simulink library "InterModuleProtocol"  (R2023b)
settings: Solver=VariableStepAuto  StartTime=0.0  StopTime=10.0  RelTol=1e-3
undefined symbols (not defined in the file or in its folder): accelerationNED, accelerationNEDXYZ, accelerationXYZ, angleOfAttack, courseOverGround, orientationQuaternion, orientationRollPitchYaw, positionLLA, positionNED, sideSlipAngle, speedOverGround, velocityNED, velocityNEDUVW, velocityPQR, velocityUVW
libraries: $bdroot x10
(part 1 of 3)
settings Model: Creator=Scythe  LastModifiedBy=Scythe
settings SolverCC: AlgebraicLoopSolver=TrustRegion
settings DataIOCC: ReturnWorkspaceOutputs=off
settings OptimizationCC: ReuseModelBlockBuffer=off
settings DebuggingCC: UnconnectedInputMsg=warning  UnconnectedOutputMsg=warning  UnconnectedLineMsg=warning  ArithmeticOperatorsInVariantConditions=warning
settings ModelReferenceCC: EnableRefExpFcnMdlSchedulingChecks=on
settings SFSimCC: CustomCodeUndefinedFunction=UseInterfaceOnly
settings RTWCC: DLArmComputeVersion=19.05

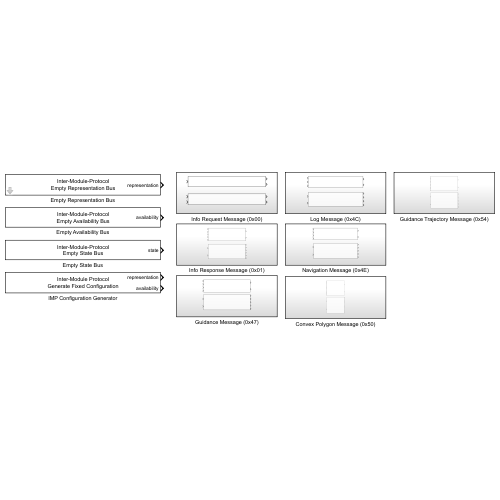
[thumbnail: Simulink's stored preview of the top-level diagram]
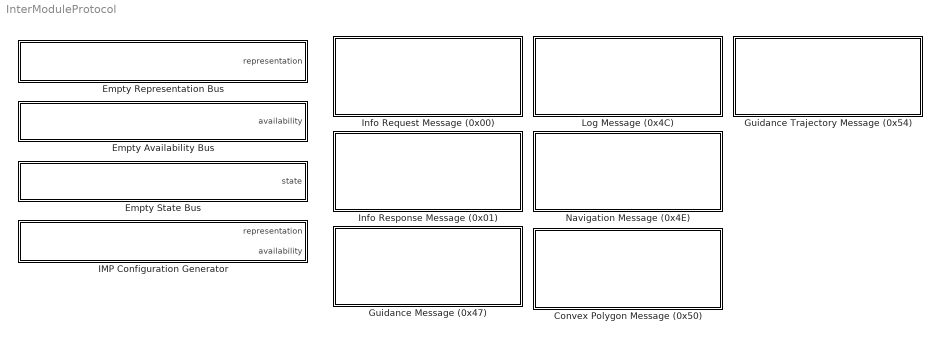
== system InterModuleProtocol ==
  Convex Polygon Message (0x50) : Subsystem
  Empty Availability Bus : Subsystem
      mask help: Create an empty availability bus for the Inter-Module Protocol (IMP). All values inside the bus are zero.
      mask DialogControl DescGroupVar Prompt: Empty Availability Bus
      mask Display: disp('Inter-Module-Protocol\nEmpty Availability Bus');
  Empty Representation Bus : Subsystem
      mask help: Create an empty representation bus for the Inter-Module Protocol (IMP). All values inside the bus are zero.
      mask DialogControl DescGroupVar Prompt: Empty Representation Bus
      mask Display: disp('Inter-Module-Protocol\nEmpty Representation Bus');
  Empty State Bus : Subsystem
      mask help: Create an empty state bus for the Inter-Module Protocol (IMP). All values inside the bus are zero. However, the scalar part of the quaternion is set to one.
      mask DialogControl DescGroupVar Prompt: Empty State Bus
      mask Display: disp('Inter-Module-Protocol\nEmpty State Bus');
  Guidance Message (0x47) : Subsystem
  Guidance Trajectory Message (0x54) : Subsystem
  IMP Configuration Generator : Subsystem  mask{positionLLAAvailability=0 DoF - none, positionLLARepresentation=8 bytes (double), positionNEDAvailability=0 DoF - none, positionNEDRepresentation=8 bytes (double), orientationQuaternionAvailability=0 DoF - none, orientationQuaternionRepresentation=8 bytes (double), orientationRPYAvailability=0 DoF - none, orientationRPYRepresentation=8 bytes (double), velocityNEDUVWAvailabilityE=0 DoF - none, velocityNEDUVWAvailabilityB=0 DoF - none, velocityNEDUVWRepresentation=8 bytes (double), velocityPQRAvailability=0 DoF - none, velocityPQRRepresentation=8 bytes (double), accelerationNEDXYZAvailabilityE=0 DoF - none, accelerationNEDXYZAvailabilityB=0 DoF - none, accelerationNEDXYZRepresentation=8 bytes (double), courseOverGroundAvailability=0 - disable, courseOverGroundRepresentation=8 bytes (double), speedOverGroundAvailability=0 - disable, speedOverGroundRepresentation=8 bytes (double), angleOfAttackAvailability=0 - disable, angleOfAttackRepresentation=8 bytes (double), sideSlipAngleAvailability=0 - disable, sideSlipAngleRepresentation=8 bytes (double)}
      mask prompts: positionLLAAvailability "Position (latitude, longitude, altitude):"; positionLLARepresentation ""; positionNEDAvailability "Position (NED):"; positionNEDRepresentation ""; orientationQuaternionAvailability "Orientation (quaternion):"; orientationQuaternionRepresentation ""; orientationRPYAvailability "Orientation (roll, pitch, yaw):"; orientationRPYRepresentation ""; velocityNEDUVWAvailabilityE "Velocity (NED, uvw):"; velocityPQRAvailability "Velocity (pqr):"; velocityPQRRepresentation ""; accelerationNEDXYZAvailabilityE "Acceleration (NED, XYZ):"; courseOverGroundAvailability "Course over ground:"; courseOverGroundRepresentation ""; speedOverGroundAvailability "Speed over ground:"; speedOverGroundRepresentation ""; angleOfAttackAvailability "Angle of attack:"; angleOfAttackRepresentation ""; sideSlipAngleAvailability "Side slip angle:"; sideSlipAngleRepresentation ""
      mask help: Generate a fixed configuration (representation and availability) to be used for encoding messages like navigation and guidance messages. The configuration is used to encode a variable-data message. For each value in a message, select the degree of freedom (DoF) and the data type representation to be encoded.
      mask TypeOptions positionLLAAvailability: 0 DoF - none | 1 DoF - alt | 2 DoF - lat, lon | 3 DoF - lat, lon, alt
      mask TypeOptions positionLLARepresentation: 4 bytes (int32, float) | 8 bytes (double)
      mask TypeOptions positionNEDAvailability: 0 DoF - none | 1 DoF - down | 2 DoF - north, east | 3 DoF - north, east, down
      mask TypeOptions positionNEDRepresentation: 4 bytes (float) | 8 bytes (double)
      mask TypeOptions orientationQuaternionAvailability: 0 DoF - none | 3 DoF - qw, qx, qy, qz
      mask TypeOptions orientationQuaternionRepresentation: 4 bytes (int32) | 8 bytes (double)
      mask TypeOptions orientationRPYAvailability: 0 DoF - none | 1 DoF - yaw | 2 DoF - roll, pitch | 3 DoF - roll, pitch, yaw
      mask TypeOptions orientationRPYRepresentation: 4 bytes (int32) | 8 bytes (double)
      mask TypeOptions velocityNEDUVWAvailabilityE: 0 DoF - none | 1 DoF - down | 2 DoF - north, east | 3 DoF - north, east, down
      mask TypeOptions velocityNEDUVWAvailabilityB: 0 DoF - none | 1 DoF - w | 2 DoF - u, v | 3 DoF - u, v, w
      mask TypeOptions velocityNEDUVWRepresentation: 4 bytes (float) | 8 bytes (double)
      mask TypeOptions velocityPQRAvailability: 0 DoF - none | 1 DoF - r | 2 DoF - p, q | 3 DoF - p, q, r
      mask TypeOptions velocityPQRRepresentation: 4 bytes (float) | 8 bytes (double)
      mask TypeOptions accelerationNEDXYZAvailabilityE: 0 DoF - none | 1 DoF - down | 2 DoF - north, east | 3 DoF - north, east, down
      mask TypeOptions accelerationNEDXYZAvailabilityB: 0 DoF - none | 1 DoF - Z | 2 DoF - X, Y | 3 DoF - X, Y, Z
      mask TypeOptions accelerationNEDXYZRepresentation: 4 bytes (float) | 8 bytes (double)
      mask TypeOptions courseOverGroundAvailability: 0 - disable | 1 - enable
      mask TypeOptions courseOverGroundRepresentation: 4 bytes (int32) | 8 bytes (double)
      mask TypeOptions speedOverGroundAvailability: 0 - disable | 1 - enable
      mask TypeOptions speedOverGroundRepresentation: 4 bytes (float) | 8 bytes (double)
      mask TypeOptions angleOfAttackAvailability: 0 - disable | 1 - enable
      mask TypeOptions angleOfAttackRepresentation: 4 bytes (int32) | 8 bytes (double)
      mask TypeOptions sideSlipAngleAvailability: 0 - disable | 1 - enable
      mask TypeOptions sideSlipAngleRepresentation: 4 bytes (int32) | 8 bytes (double)
      mask DialogControl DescGroupVar Prompt: Generate Fixed Configuration
      mask DialogControl ParameterGroupVar Prompt: Configuration
      mask Display: disp('Inter-Module Protocol\nGenerate Fixed Configuration');
  Info Request Message (0x00) : Subsystem
  Info Response Message (0x01) : Subsystem
  Log Message (0x4C) : Subsystem
  Navigation Message (0x4E) : Subsystem

== system InterModuleProtocol/Convex Polygon Message (0x50) ==
  Decode Convex Polygon Message : Subsystem  mask{maxNumPolygons=10}
      mask prompts: maxNumPolygons "Maximum number of polygons:"
      mask help:
      | Decode a convex polygon message (Inter-Module Protocol).<br><br>
      |
      | <b>numDecodedBytes</b><br>Number of decoded bytes (negative value if error occurred).<br><br>
      | <b>timestampUTC</b><br>UTC second of the day.<br><br>
      | <b>maxSegmentIndex</b><br>The maximum zero-based segment index that indicates the last message segment. That is, the maximum number of polgon messages belonging to a polygon dataset is (maxSegmentIndex + 1).<br><br>
      | <b>segmentIndex</b><br>The current zero-based segment index for this message.<br><br>
      | <b>originLLA</b><br>Latitude [rad], longitude [rad] and altitude [m] of the origin.<br><br>
      | <b>polygons</b><br>A 2-by-255-by-np matrix containing the vertices for all polygons (column-major order) with np being the maximum number of polygons. A vertex consists of two elements (x and y).<br><br>
      | <b>numVertices</b><br>An np-by-1 vector containing the unique IDs for all polygons in the polygon matrix.<br><br>
      | <b>polygonIDs</b><br>An np-by-1 vector containing the unique IDs for all polygons in the polygon matrix with np being the maximum number of polygons.<br><br>
      | <b>classifications</b><br>An np-by-1 vector containing the classifications for all polygons in the polygon matrix with np being the maximum number of polygons.<br><br>
      | <b>velocitiesNorth</b><br>An np-by-1 vector containing the north velocities in meters per second for all polygons in the polygon matrix with np being the maximum number of polygons. All velocities of a polygon refer to the mean value of all vertices of this polygon.<br><br>
      | <b>velocitiesEast</b><br>An np-by-1 vector containing the east velocities in meters per second for all polygons in the polygon matrix with np being the maximum number of polygons. All velocities of a polygon refer to the mean value of all vertices of this polygon.<br><br>
      | <b>velocitiesYawRate</b><br>An np-by-1 vector containing the rotational rates of turn in radians per second for all polygons in the polygon matrix with np being the maximum number of polygons. All velocities of a polygon refer to the mean value of all vertices of this polygon.<br><br>
      | <b>numPolygons</b><br>The number of decoded polygons.
      mask Help: eval('IMP_OpenDocumentation(''#ConvexPolygonMessage'');');
      mask DialogControl DescGroupVar Prompt: Decode Convex Polygon Message
      mask Display: disp('Inter-Module-Protocol\nDecode Convex Polygon Message');
  Encode Convex Polygon Message : Subsystem  mask{outBufferSize=1024, maxNumPolygons=10}
      mask prompts: outBufferSize "Output buffer size:"; maxNumPolygons "Maximum number of polygons:"
      mask help:
      | Encode a convex polygon message (Inter-Module Protocol).<br><br>
      |
      | <b>timestampUTC</b><br>UTC second of the day.<br><br>
      | <b>maxSegmentIndex</b><br>The maximum zero-based segment index that indicates the last message segment. That is, the maximum number of polgon messages belonging to a polygon dataset is (maxSegmentIndex + 1).<br><br>
      | <b>segmentIndex</b><br>The current zero-based segment index for this message.<br><br>
      | <b>originLLA</b><br>Latitude [rad], longitude [rad] and altitude [m] of the origin.<br><br>
      | <b>polygons</b><br>A 2-by-255-by-np matrix containing the vertices for all polygons (column-major order) with np being the maximum number of polygons. A vertex consists of two elements (x and y).<br><br>
      | <b>numVertices</b><br>An np-by-1 vector containing the actual number of vertices per polygon in the polygon matrix.<br><br>
      | <b>polygonIDs</b><br>An np-by-1 vector containing the unique IDs for all polygons in the polygon matrix with np being the maximum number of polygons.<br><br>
      | <b>classifications</b><br>An np-by-1 vector containing the classifications for all polygons in the polygon matrix with np being the maximum number of polygons.<br><br>
      | <b>velocitiesNorth</b><br>An np-by-1 vector containing the north velocities in meters per second for all polygons in the polygon matrix with np being the maximum number of polygons. All velocities of a polygon refer to the mean value of all vertices of this polygon.<br><br>
      | <b>velocitiesEast</b><br>An np-by-1 vector containing the east velocities in meters per second for all polygons in the polygon matrix with np being the maximum number of polygons. All velocities of a polygon refer to the mean value of all vertices of this polygon.<br><br>
      | <b>velocitiesYawRate</b><br>An np-by-1 vector containing the rotational rates of turn in radians per second for all polygons in the polygon matrix with np being the maximum number of polygons. All velocities of a polygon refer to the mean value of all vertices of this polygon.<br><br>
      | <b>numPolygons</b><br>The number of polygons to be used for encoding.
      mask Help: eval('IMP_OpenDocumentation(''#ConvexPolygonMessage'');');
      mask DialogControl DescGroupVar Prompt: Encode Convex Polygon Message
      mask Display: disp('Inter-Module-Protocol\nEncode Convex Polygon Message');

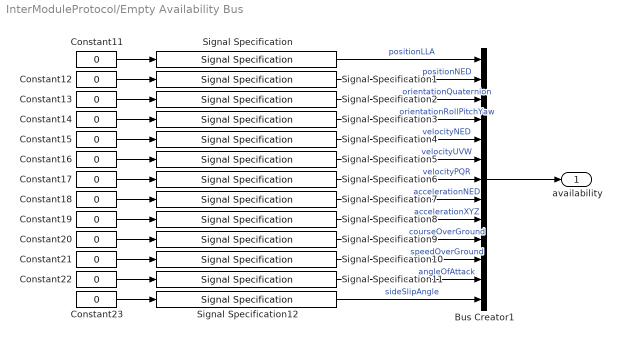
== system InterModuleProtocol/Empty Availability Bus ==
  Bus Creator1 : BusCreator  Inputs=13
  Constant{11..23} (13 alike) : Constant  Value=0  OutDataTypeStr=uint8
  Signal Specification{,1..12} (13 alike) : SignalSpecification  OutDataTypeStr=uint8  Dimensions=1
  availability : Outport  VectorParamsAs1DForOutWhenUnconnected=off
  wires:
  Signal Specification10/1 -> Bus Creator1/11  "speedOverGround"
  Signal Specification3/1 -> Bus Creator1/4  "orientationRollPitchYaw"
  Signal Specification4/1 -> Bus Creator1/5  "velocityNED"
  Signal Specification12/1 -> Bus Creator1/13  "sideSlipAngle"
  Bus Creator1/1 -> availability/1
  Signal Specification1/1 -> Bus Creator1/2  "positionNED"
  Signal Specification9/1 -> Bus Creator1/10  "courseOverGround"
  Signal Specification5/1 -> Bus Creator1/6  "velocityUVW"
  Signal Specification6/1 -> Bus Creator1/7  "velocityPQR"
  Signal Specification2/1 -> Bus Creator1/3  "orientationQuaternion"
  Signal Specification/1 -> Bus Creator1/1  "positionLLA"
  Signal Specification7/1 -> Bus Creator1/8  "accelerationNED"
  Signal Specification8/1 -> Bus Creator1/9  "accelerationXYZ"
  Signal Specification11/1 -> Bus Creator1/12  "angleOfAttack"
  Constant11/1 -> Signal Specification/1
  Constant12/1 -> Signal Specification1/1
  Constant13/1 -> Signal Specification2/1
  Constant14/1 -> Signal Specification3/1
  Constant15/1 -> Signal Specification4/1
  Constant16/1 -> Signal Specification5/1
  Constant23/1 -> Signal Specification12/1
  Constant22/1 -> Signal Specification11/1
  Constant21/1 -> Signal Specification10/1
  Constant20/1 -> Signal Specification9/1
  Constant19/1 -> Signal Specification8/1
  Constant18/1 -> Signal Specification7/1
  Constant17/1 -> Signal Specification6/1

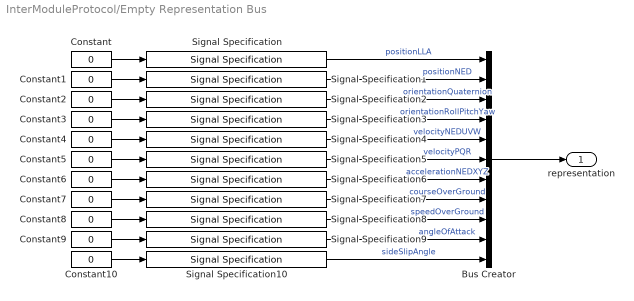
== system InterModuleProtocol/Empty Representation Bus ==
  Bus Creator : BusCreator  Inputs=11
  Constant{,1..10} (11 alike) : Constant  Value=0  OutDataTypeStr=uint8
  Signal Specification{,1..10} (11 alike) : SignalSpecification  OutDataTypeStr=uint8  Dimensions=1
  representation : Outport  VectorParamsAs1DForOutWhenUnconnected=off
  wires:
  Signal Specification10/1 -> Bus Creator/11  "sideSlipAngle"
  Signal Specification1/1 -> Bus Creator/2  "positionNED"
  Signal Specification8/1 -> Bus Creator/9  "speedOverGround"
  Bus Creator/1 -> representation/1
  Signal Specification9/1 -> Bus Creator/10  "angleOfAttack"
  Signal Specification7/1 -> Bus Creator/8  "courseOverGround"
  Signal Specification6/1 -> Bus Creator/7  "accelerationNEDXYZ"
  Signal Specification4/1 -> Bus Creator/5  "velocityNEDUVW"
  Signal Specification5/1 -> Bus Creator/6  "velocityPQR"
  Signal Specification3/1 -> Bus Creator/4  "orientationRollPitchYaw"
  Signal Specification2/1 -> Bus Creator/3  "orientationQuaternion"
  Signal Specification/1 -> Bus Creator/1  "positionLLA"
  Constant/1 -> Signal Specification/1
  Constant1/1 -> Signal Specification1/1
  Constant2/1 -> Signal Specification2/1
  Constant3/1 -> Signal Specification3/1
  Constant4/1 -> Signal Specification4/1
  Constant5/1 -> Signal Specification5/1
  Constant6/1 -> Signal Specification6/1
  Constant7/1 -> Signal Specification7/1
  Constant8/1 -> Signal Specification8/1
  Constant9/1 -> Signal Specification9/1
  Constant10/1 -> Signal Specification10/1

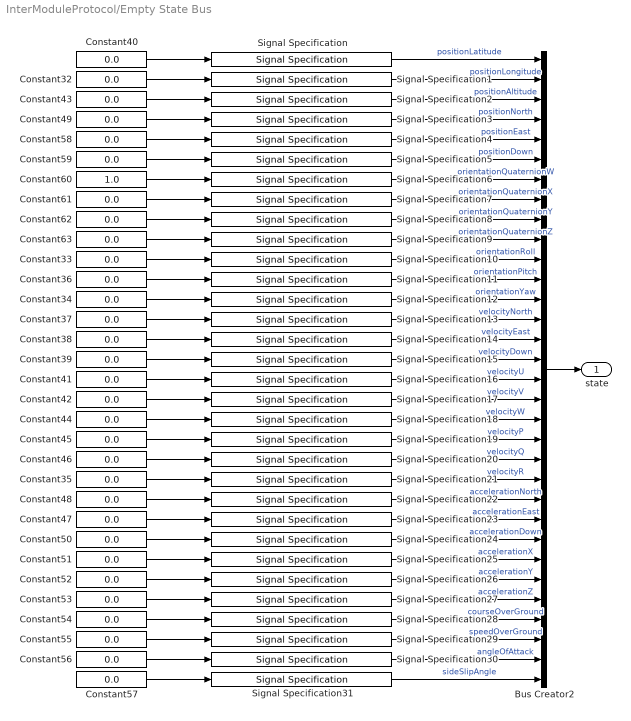
== system InterModuleProtocol/Empty State Bus ==
  Bus Creator2 : BusCreator  Inputs=32
  Constant{32..59,61..63} (31 alike) : Constant  Value=0.0
  Constant60 : Constant  Value=1.0
  Signal Specification{,1,10..12,28,30..31} (8 alike) : SignalSpecification  OutDataTypeStr=double  Unit=rad  Dimensions=1
  Signal Specification{13..18,29} (7 alike) : SignalSpecification  OutDataTypeStr=double  Unit=m/s  Dimensions=1
  Signal Specification19 : SignalSpecification  OutDataTypeStr=double  Unit=rad/s  Dimensions=1
  Signal Specification{2..5} (4 alike) : SignalSpecification  OutDataTypeStr=double  Unit=m  Dimensions=1
  Signal Specification20 : SignalSpecification  OutDataTypeStr=double  Unit=rad/s  Dimensions=1
  Signal Specification21 : SignalSpecification  OutDataTypeStr=double  Unit=rad/s  Dimensions=1
  Signal Specification{22..27} (6 alike) : SignalSpecification  OutDataTypeStr=double  Unit=m/s^2  Dimensions=1
  Signal Specification{6..9} (4 alike) : SignalSpecification  OutDataTypeStr=double  Dimensions=1
  state : Outport  VectorParamsAs1DForOutWhenUnconnected=off
  wires:
  Signal Specification29/1 -> Bus Creator2/30  "speedOverGround"
  Signal Specification2/1 -> Bus Creator2/3  "positionAltitude"
  Signal Specification8/1 -> Bus Creator2/9  "orientationQuaternionY"
  Signal Specification17/1 -> Bus Creator2/18  "velocityV"
  Bus Creator2/1 -> state/1
  Signal Specification25/1 -> Bus Creator2/26  "accelerationX"
  Signal Specification1/1 -> Bus Creator2/2  "positionLongitude"
  Signal Specification27/1 -> Bus Creator2/28  "accelerationZ"
  Signal Specification3/1 -> Bus Creator2/4  "positionNorth"
  Signal Specification12/1 -> Bus Creator2/13  "orientationYaw"
  Signal Specification18/1 -> Bus Creator2/19  "velocityW"
  Signal Specification24/1 -> Bus Creator2/25  "accelerationDown"
  Signal Specification22/1 -> Bus Creator2/23  "accelerationNorth"
  Signal Specification/1 -> Bus Creator2/1  "positionLatitude"
  Signal Specification15/1 -> Bus Creator2/16  "velocityDown"
  Signal Specification14/1 -> Bus Creator2/15  "velocityEast"
  Signal Specification10/1 -> Bus Creator2/11  "orientationRoll"
  Signal Specification26/1 -> Bus Creator2/27  "accelerationY"
  Signal Specification30/1 -> Bus Creator2/31  "angleOfAttack"
  Signal Specification6/1 -> Bus Creator2/7  "orientationQuaternionW"
  Signal Specification13/1 -> Bus Creator2/14  "velocityNorth"
  Signal Specification11/1 -> Bus Creator2/12  "orientationPitch"
  Signal Specification16/1 -> Bus Creator2/17  "velocityU"
  Signal Specification21/1 -> Bus Creator2/22  "velocityR"
  Signal Specification19/1 -> Bus Creator2/20  "velocityP"
  Signal Specification31/1 -> Bus Creator2/32  "sideSlipAngle"
  Signal Specification4/1 -> Bus Creator2/5  "positionEast"
  Signal Specification7/1 -> Bus Creator2/8  "orientationQuaternionX"
  Signal Specification5/1 -> Bus Creator2/6  "positionDown"
  Signal Specification9/1 -> Bus Creator2/10  "orientationQuaternionZ"
  Signal Specification28/1 -> Bus Creator2/29  "courseOverGround"
  Signal Specification20/1 -> Bus Creator2/21  "velocityQ"
  Signal Specification23/1 -> Bus Creator2/24  "accelerationEast"
  Constant50/1 -> Signal Specification24/1
  Constant56/1 -> Signal Specification30/1
  Constant52/1 -> Signal Specification26/1
  Constant47/1 -> Signal Specification23/1
  Constant33/1 -> Signal Specification10/1
  Constant43/1 -> Signal Specification2/1
  Constant40/1 -> Signal Specification/1
  Constant51/1 -> Signal Specification25/1
  Constant34/1 -> Signal Specification12/1
  Constant49/1 -> Signal Specification3/1
  Constant36/1 -> Signal Specification11/1
  Constant37/1 -> Signal Specification13/1
  Constant35/1 -> Signal Specification21/1
  Constant55/1 -> Signal Specification29/1
  Constant62/1 -> Signal Specification8/1
  Constant63/1 -> Signal Specification9/1
  Constant54/1 -> Signal Specification28/1
  Constant53/1 -> Signal Specification27/1
  Constant39/1 -> Signal Specification15/1
  Constant59/1 -> Signal Specification5/1
  Constant41/1 -> Signal Specification16/1
  Constant61/1 -> Signal Specification7/1
  Constant38/1 -> Signal Specification14/1
  Constant58/1 -> Signal Specification4/1
  Constant60/1 -> Signal Specification6/1
  Constant46/1 -> Signal Specification20/1
  Constant32/1 -> Signal Specification1/1
  Constant44/1 -> Signal Specification18/1
  Constant57/1 -> Signal Specification31/1
  Constant42/1 -> Signal Specification17/1
  Constant48/1 -> Signal Specification22/1
  Constant45/1 -> Signal Specification19/1

== system InterModuleProtocol/Guidance Message (0x47) ==
  Decode Guidance Message : Subsystem
      mask help:
      | Decode a guidance message (Inter-Module Protocol).<br><br>
      |
      | <b>numDecodedBytes</b><br>Number of decoded bytes (negative value if error occurred).<br><br>
      | <b>timestampUTC</b><br>UTC second of the day.<br><br>
      | <b>representation</b><br>Representation bus containing the datatype representation for the state.<br><br>
      | <b>availability</b><br>Availability bus containing the availability flags for the state.<br><br>
      | <b>state</b><br>The state bus containing the decoded values.
      mask Help: eval('IMP_OpenDocumentation(''#GuidanceMessage'');');
      mask DialogControl DescGroupVar Prompt: Decode Guidance Message
      mask Display: disp('Inter-Module-Protocol\nDecode Guidance Message');
  Encode Guidance Message : Subsystem  mask{outputBufferSize=268}
      mask prompts: outputBufferSize "Output buffer size:"
      mask help:
      | Encode a guidance message (Inter-Module Protocol).<br><br>
      |
      | <b>timestampUTC</b><br>UTC second of the day.<br><br>
      | <b>representation</b><br>The representation bus containing the data type representation for the state.
      | <br><br>
      |
      | <b>availability</b><br>The availability bus containing the availability flags for the state.
      | <br><br>
      |
      | <b>state</b><br>The state bus containing the values to be encoded.
      mask Help: eval('IMP_OpenDocumentation(''#GuidanceMessage'');');
      mask DialogControl DescGroupVar Prompt: Encode Guidance Message
      mask DialogControl Container2 Prompt: Parameters
      mask Display: disp('Inter-Module-Protocol\nEncode Guidance Message');

== system InterModuleProtocol/Guidance Trajectory Message (0x54) ==
  Decode Guidance Trajectory Message : Subsystem  mask{maxNumPoints=10}
      mask prompts: maxNumPoints "Maximum number of points:"
      mask help:
      | Decode a guidance trajectory message (Inter-Module Protocol).<br><br>
      |
      | <b>numDecodedBytes</b><br>Number of decoded bytes (negative value if error occurred).<br><br>
      | <b>timestampUTC</b><br>UTC second of the day.<br><br>
      | <b>startTimeYearUTC</b><br>Start time for the trajectory: year (UTC).<br><br>
      | <b>startTimeMonthUTC</b><br>Start time for the trajectory: month (UTC), range [1, 12].<br><br>
      | <b>startTimeDayUTC</b><br>Start time for the trajectory: day (UTC), range [1, 31].<br><br>
      | <b>startTimeSecondsUTC</b><br>Start time for the trajectory: seconds of the day (UTC).<br><br>
      | <b>deltaTime</b><br>Time difference from one state point to another in seconds. If this value is set to zero, then each point indicates a waypoint.<br><br>
      | <b>representation</b><br>Representation bus containing the datatype representation for a point.<br><br>
      | <b>availability</b><br>Availability bus containing the availability flags for a point.<br><br>
      | <b>points</b><br>32-by-N matrix containing N state vectors. N is the maximum number of points. Each column of the matrix is as follows:
      | <br>[0]: positionLatitude (rad)
      | <br>[1]: positionLongitude (rad)
      | <br>[2]: positionAltitude (m)
      | <br>[3]: positionNorth (m)
      | <br>[4]: positionEast (m)
      | <br>[5]: positionDown (m)
      | <br>[6]: orientationQuaternionW
      | <br>[7]: orientationQuaternionX
      | <br>[8]: orientationQuaternionY
      | <br>[9]: orientationQuaternionZ
      | <br>[10]: orientationRoll (rad)
      | <br>[11]: orientationPitch (rad)
      | <br>[12]: orientationYaw (rad)
      | <br>[13]: velocityNorth (m/s)
      | <br>[14]: velocityEast (m/s)
      | <br>[15]: velocityDown (m/s)
      | <br>[16]: velocityU (m/s)
      | <br>[17]: velocityV (m/s)
      | <br>[18]: velocityW (m/s)
      | <br>[19]: velocityP (rad/s)
      | <br>[20]: velocityQ (rad/s)
      | <br>[21]: velocityR (rad/s)
      | <br>[22]: accelerationNorth (m/(s*s))
      | <br>[23]: accelerationEast (m/(s*s))
      | <br>[24]: accelerationDown (m/(s*s))
      | <br>[25]: accelerationX (m/(s*s))
      | <br>[26]: accelerationY (m/(s*s))
      | <br>[27]: accelerationZ (m/(s*s))
      | <br>[28]: courseOverGround (rad)
      | <br>[29]: speedOverGround (m/s)
      | <br>[30]: angleOfAttack (rad)
      | <br>[31]: sideSlipAngle (rad)
      | <br><br>
      | <b>numPoints</b><br>Actual number of decoded points inside the output matrix.
      mask Help: eval('IMP_OpenDocumentation(''#GuidanceTrajectoryMessage'');');
      mask DialogControl DescGroupVar Prompt: Decode Guidance Trajectory Message
      mask Display: disp('Inter-Module-Protocol\nDecode Guidance Trajectory Message');
  Encode Guidance Trajectory Message : Subsystem  mask{maxNumPoints=10, outputBufferSize=1024}
      mask prompts: maxNumPoints "Maximum number of points:"; outputBufferSize "Output buffer size:"
      mask help:
      | Encode a guidance trajectory message (Inter-Module Protocol).<br><br>
      |
      | <b>timestampUTC</b><br>UTC second of the day.<br><br>
      | <b>startTimeYearUTC</b><br>Start time for the trajectory: year (UTC).<br><br>
      | <b>startTimeMonthUTC</b><br>Start time for the trajectory: month (UTC), range [1, 12].<br><br>
      | <b>startTimeDayUTC</b><br>Start time for the trajectory: day (UTC), range [1, 31].<br><br>
      | <b>startTimeSecondsUTC</b><br>Start time for the trajectory: seconds of the day (UTC).<br><br>
      | <b>deltaTime</b><br>Time difference from one state point to another in seconds. If this value is set to zero, then each point indicates a waypoint.<br><br>
      | <b>representation</b><br>The representation bus containing the data type representation for a point.<br><br>
      | <b>availability</b><br>The availability bus containing the availability flags for a point.<br><br>
      | <b>points</b><br>32-by-N matrix containing N state vectors. N is the number of points. Each column of the matrix is as follows:
      | <br>[0]: positionLatitude (rad)
      | <br>[1]: positionLongitude (rad)
      | <br>[2]: positionAltitude (m)
      | <br>[3]: positionNorth (m)
      | <br>[4]: positionEast (m)
      | <br>[5]: positionDown (m)
      | <br>[6]: orientationQuaternionW
      | <br>[7]: orientationQuaternionX
      | <br>[8]: orientationQuaternionY
      | <br>[9]: orientationQuaternionZ
      | <br>[10]: orientationRoll (rad)
      | <br>[11]: orientationPitch (rad)
      | <br>[12]: orientationYaw (rad)
      | <br>[13]: velocityNorth (m/s)
      | <br>[14]: velocityEast (m/s)
      | <br>[15]: velocityDown (m/s)
      | <br>[16]: velocityU (m/s)
      | <br>[17]: velocityV (m/s)
      | <br>[18]: velocityW (m/s)
      | <br>[19]: velocityP (rad/s)
      | <br>[20]: velocityQ (rad/s)
      | <br>[21]: velocityR (rad/s)
      | <br>[22]: accelerationNorth (m/(s*s))
      | <br>[23]: accelerationEast (m/(s*s))
      | <br>[24]: accelerationDown (m/(s*s))
      | <br>[25]: accelerationX (m/(s*s))
      | <br>[26]: accelerationY (m/(s*s))
      | <br>[27]: accelerationZ (m/(s*s))
      | <br>[28]: courseOverGround (rad)
      | <br>[29]: speedOverGround (m/s)
      | <br>[30]: angleOfAttack (rad)
      | <br>[31]: sideSlipAngle (rad)
      mask Help: eval('IMP_OpenDocumentation(''#GuidanceTrajectoryMessage'');');
      mask DialogControl DescGroupVar Prompt: Encode Guidance Trajectory Message
      mask Display: disp('Inter-Module-Protocol\nEncode Guidance Trajectory Message');

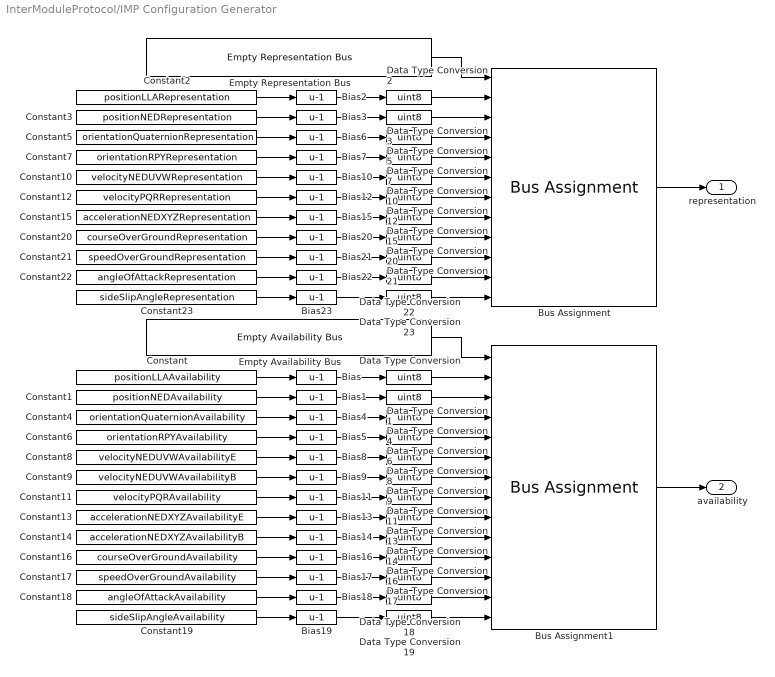
== system InterModuleProtocol/IMP Configuration Generator ==
  Bias{,1..23} (24 alike) : Bias  Bias=-1  SaturateOnIntegerOverflow=off
  Bus Assignment : BusAssignment  AssignedSignals=positionLLA,positionNED,orientationQuaternion,orientationRollPitchYaw,velocityNEDUVW,velocityPQR,accelerationNEDXYZ,courseOverGround,speedOverGround,angleOfAttack,sideSlipAngle
  Bus Assignment1 : BusAssignment  AssignedSignals=positionLLA,positionNED,orientationQuaternion,orientationRollPitchYaw,velocityNED,velocityUVW,velocityPQR,accelerationNED,accelerationXYZ,courseOverGround,speedOverGround,angleOfAttack,sideSlipAngle
  Constant : Constant  Value=positionLLAAvailability
  Constant1 : Constant  Value=positionNEDAvailability
  Constant10 : Constant  Value=velocityNEDUVWRepresentation
  Constant11 : Constant  Value=velocityPQRAvailability
  Constant12 : Constant  Value=velocityPQRRepresentation
  Constant13 : Constant  Value=accelerationNEDXYZAvailabilityE
  Constant14 : Constant  Value=accelerationNEDXYZAvailabilityB
  Constant15 : Constant  Value=accelerationNEDXYZRepresentation
  Constant16 : Constant  Value=courseOverGroundAvailability
  Constant17 : Constant  Value=speedOverGroundAvailability
  Constant18 : Constant  Value=angleOfAttackAvailability
  Constant19 : Constant  Value=sideSlipAngleAvailability
  Constant2 : Constant  Value=positionLLARepresentation
  Constant20 : Constant  Value=courseOverGroundRepresentation
  Constant21 : Constant  Value=speedOverGroundRepresentation
  Constant22 : Constant  Value=angleOfAttackRepresentation
  Constant23 : Constant  Value=sideSlipAngleRepresentation
  Constant3 : Constant  Value=positionNEDRepresentation
  Constant4 : Constant  Value=orientationQuaternionAvailability
  Constant5 : Constant  Value=orientationQuaternionRepresentation
  Constant6 : Constant  Value=orientationRPYAvailability
  Constant7 : Constant  Value=orientationRPYRepresentation
  Constant8 : Constant  Value=velocityNEDUVWAvailabilityE
  Constant9 : Constant  Value=velocityNEDUVWAvailabilityB
  Data Type Conversion{,1..23} (24 alike) : DataTypeConversion  OutDataTypeStr=uint8  SaturateOnIntegerOverflow=off  RndMeth=Floor
  Empty Availability Bus : $bdroot/Empty Availability Bus
  Empty Representation Bus : $bdroot/Empty Representation Bus
  representation : Outport
  availability : Outport  Port=2
  wires:
  Bias20/1 -> Data Type Conversion20/1
  Constant20/1 -> Bias20/1
  Constant21/1 -> Bias21/1
  Bias21/1 -> Data Type Conversion21/1
  Bias22/1 -> Data Type Conversion22/1
  Constant22/1 -> Bias22/1
  Constant23/1 -> Bias23/1
  Bias23/1 -> Data Type Conversion23/1
  Bias19/1 -> Data Type Conversion19/1
  Constant19/1 -> Bias19/1
  Constant18/1 -> Bias18/1
  Bias18/1 -> Data Type Conversion18/1
  Bias17/1 -> Data Type Conversion17/1
  Constant17/1 -> Bias17/1
  Constant16/1 -> Bias16/1
  Bias16/1 -> Data Type Conversion16/1
  Constant15/1 -> Bias15/1
  Bias15/1 -> Data Type Conversion15/1
  Constant13/1 -> Bias13/1
  Bias13/1 -> Data Type Conversion13/1
  Bias14/1 -> Data Type Conversion14/1
  Constant14/1 -> Bias14/1
  Bias12/1 -> Data Type Conversion12/1
  Constant12/1 -> Bias12/1
  Bias11/1 -> Data Type Conversion11/1
  Constant11/1 -> Bias11/1
  Constant10/1 -> Bias10/1
  Bias10/1 -> Data Type Conversion10/1
  Constant9/1 -> Bias9/1
  Bias9/1 -> Data Type Conversion9/1
  Bias8/1 -> Data Type Conversion8/1
  Constant8/1 -> Bias8/1
  Bias7/1 -> Data Type Conversion7/1
  Constant7/1 -> Bias7/1
  Constant6/1 -> Bias5/1
  Bias5/1 -> Data Type Conversion6/1
  Constant5/1 -> Bias6/1
  Bias6/1 -> Data Type Conversion5/1
  Bias4/1 -> Data Type Conversion4/1
  Constant4/1 -> Bias4/1
  Constant2/1 -> Bias2/1
  Bias2/1 -> Data Type Conversion2/1
  Bias3/1 -> Data Type Conversion3/1
  Constant3/1 -> Bias3/1
  Constant1/1 -> Bias1/1
  Bias1/1 -> Data Type Conversion1/1
  Bias/1 -> Data Type Conversion/1
  Constant/1 -> Bias/1
  Empty Representation Bus/1 -> Bus Assignment/1
  Bus Assignment/1 -> representation/1
  Empty Availability Bus/1 -> Bus Assignment1/1
  Bus Assignment1/1 -> availability/1
  Data Type Conversion/1 -> Bus Assignment1/2
  Data Type Conversion1/1 -> Bus Assignment1/3
  Data Type Conversion4/1 -> Bus Assignment1/4
  Data Type Conversion6/1 -> Bus Assignment1/5
  Data Type Conversion8/1 -> Bus Assignment1/6
  Data Type Conversion9/1 -> Bus Assignment1/7
  Data Type Conversion11/1 -> Bus Assignment1/8
  Data Type Conversion13/1 -> Bus Assignment1/9
  Data Type Conversion14/1 -> Bus Assignment1/10
  Data Type Conversion16/1 -> Bus Assignment1/11
  Data Type Conversion17/1 -> Bus Assignment1/12
  Data Type Conversion18/1 -> Bus Assignment1/13
  Data Type Conversion19/1 -> Bus Assignment1/14
  Data Type Conversion3/1 -> Bus Assignment/3
  Data Type Conversion12/1 -> Bus Assignment/7
  Data Type Conversion22/1 -> Bus Assignment/11
  Data Type Conversion2/1 -> Bus Assignment/2
  Data Type Conversion5/1 -> Bus Assignment/4
  Data Type Conversion10/1 -> Bus Assignment/6
  Data Type Conversion21/1 -> Bus Assignment/10
  Data Type Conversion23/1 -> Bus Assignment/12
  Data Type Conversion7/1 -> Bus Assignment/5
  Data Type Conversion20/1 -> Bus Assignment/9
  Data Type Conversion15/1 -> Bus Assignment/8

== system InterModuleProtocol/Info Request Message (0x00) ==
  Decode Info Request Message : Subsystem
      mask help:
      | Decode an info request message (Inter-Module Protocol).<br><br>
      |
      | <b>numDecodedBytes</b><br>Number of decoded bytes (negative value if error occurred).<br><br>
      | <b>timestampUTC</b><br>UTC second of the day.
      mask Help: eval('IMP_OpenDocumentation(''#InfoRequestMessage'');');
      mask DialogControl DescGroupVar Prompt: Decode Info Request Message
      mask Display: disp('Inter-Module-Protocol\nDecode Info Request Message');
  Encode Info Request Message : Subsystem  mask{outputBufferSize=8}
      mask prompts: outputBufferSize "Output buffer size:"
      mask help:
      | Encode an info request message (Inter-Module Protocol).<br><br>
      |
      | <b>timestampUTC</b><br>UTC second of the day.
      mask Help: eval('IMP_OpenDocumentation(''#InfoRequestMessage'');');
      mask DialogControl DescGroupVar Prompt: Encode Info Request Message
      mask DialogControl Container2 Prompt: Parameters
      mask Display: disp('Inter-Module-Protocol\nEncode Info Request Message');

== system InterModuleProtocol/Info Response Message (0x01) ==
  Decode Info Response Message : Subsystem  mask{maxTextLength=255}
      mask prompts: maxTextLength "Maximum output text length (for both textVehicleName and textDescription):"
      mask help:
      | Decode an info response message (Inter-Module Protocol).<br><br>
      |
      | <b>numDecodedBytes</b><br>Number of decoded bytes (negative value if error occurred).<br><br>
      | <b>timestampUTC</b><br>UTC second of the day.<br><br>
      | <b>cuboidDimension</b><br>3-by-1 vector: dimension of the default vehicle cuboid in meters (body-frame).<br><br>
      | <b>cuboidOffset</b><br>3-by-1 vector: offset from body-frame origin to cuboid in meters (body-frame).<br><br>
      | <b>textVehicleName</b><br>The vehicle name text string.<br><br>
      | <b>textDescription</b><br>The optional description text string.
      mask Help: eval('IMP_OpenDocumentation(''#InfoResponseMessage'');');
      mask DialogControl DescGroupVar Prompt: Decode Info Response Message
      mask Display: disp('Inter-Module-Protocol\nDecode Info Respose Message');
  Encode Info Response Message : Subsystem  mask{maxTextLength=255, outputBufferSize=1024}
      mask prompts: maxTextLength "Maximum input text length (for both textVehicleName and textDescription):"; outputBufferSize "Output buffer size:"
      mask help:
      | Encode an info response message (Inter-Module Protocol).<br><br>
      |
      | <b>timestampUTC</b><br>UTC second of the day.<br><br>
      | <b>cuboidDimension</b><br>3-by-1 vector: dimension of the default vehicle cuboid in meters (body-frame).<br><br>
      | <b>cuboidOffset</b><br>3-by-1 vector: offset from body-frame origin to cuboid in meters (body-frame).<br><br>
      | <b>textVehicleName</b><br>The vehicle name text string to be encoded.<br><br>
      | <b>textDescription</b><br>The optional description text string to be encoded.
      mask Help: eval('IMP_OpenDocumentation(''#InfoResponseMessage'');');
      mask DialogControl DescGroupVar Prompt: Encode Info Response Message
      mask Display: disp('Inter-Module-Protocol\nEncode Info Respose Message');

== system InterModuleProtocol/Log Message (0x4C) ==
  Decode Log Message : Subsystem  mask{maxTextLength=255}
      mask prompts: maxTextLength "Maximum output text length:"
      mask help:
      | Decode a log message (Inter-Module Protocol).<br><br>
      |
      | <b>numDecodedBytes</b><br>Number of decoded bytes (negative value if error occurred).<br><br>
      | <b>timestampUTC</b><br>UTC second of the day.<br><br>
      | <b>color</b><br>3-by-1 vector containing the color components (red, green, blue).<br><br>
      | <b>text</b><br>The decoded text string.
      mask Help: eval('IMP_OpenDocumentation(''#LogMessage'');');
      mask DialogControl DescGroupVar Prompt: Decode Log Message
      mask Display: disp('Inter-Module-Protocol\nDecode Log Message');
  Encode Log Message : Subsystem  mask{maxTextLength=255, outputBufferSize=1024}
      mask prompts: maxTextLength "Maximum input text length:"; outputBufferSize "Output buffer size:"
      mask help:
      | Encode a log message (Inter-Module Protocol).<br><br>
      |
      | <b>timestampUTC</b><br>UTC second of the day.<br><br>
      | <b>color</b><br>3-by-1 vector containing the color components (red, green, blue).<br><br>
      | <b>text</b><br>The text string to be encoded.
      mask Help: eval('IMP_OpenDocumentation(''#LogMessage'');');
      mask DialogControl DescGroupVar Prompt: Encode Log Message
      mask Display: disp('Inter-Module-Protocol\nEncode Log Message');

== system InterModuleProtocol/Navigation Message (0x4E) ==
  Decode Navigation Message : Subsystem
      mask help:
      | Decode a navigation message (Inter-Module Protocol).<br><br>
      |
      | <b>numDecodedBytes</b><br>Number of decoded bytes (negative value if error occurred).<br><br>
      | <b>timestampUTC</b><br>UTC second of the day.<br><br>
      | <b>representation</b><br>Representation bus containing the datatype representation for the state.<br><br>
      | <b>availability</b><br>Availability bus containing the availability flags for the state.<br><br>
      | <b>state</b><br>The state bus containing the decoded values.
      mask Help: eval('IMP_OpenDocumentation(''#NavigationMessage'');');
      mask DialogControl DescGroupVar Prompt: Decode Navigation Message
      mask Display: disp('Inter-Module-Protocol\nDecode Navigation Message');
  Encode Navigation Message : Subsystem  mask{outputBufferSize=268}
      mask prompts: outputBufferSize "Output buffer size:"
      mask help:
      | Encode a navigation message (Inter-Module Protocol).<br><br>
      |
      | <b>timestampUTC</b><br>UTC second of the day.<br><br>
      | <b>representation</b><br>The representation bus containing the data type representation for the state.<br><br>
      | <b>availability</b><br>The availability bus containing the availability flags for the state.<br><br>
      | <b>state</b><br>The state bus containing the values to be encoded.
      mask Help: eval('IMP_OpenDocumentation(''#NavigationMessage'');');
      mask DialogControl DescGroupVar Prompt: Encode Navigation Message
      mask DialogControl Container2 Prompt: Parameters
      mask Display: disp('Inter-Module-Protocol\nEncode Navigation Message');

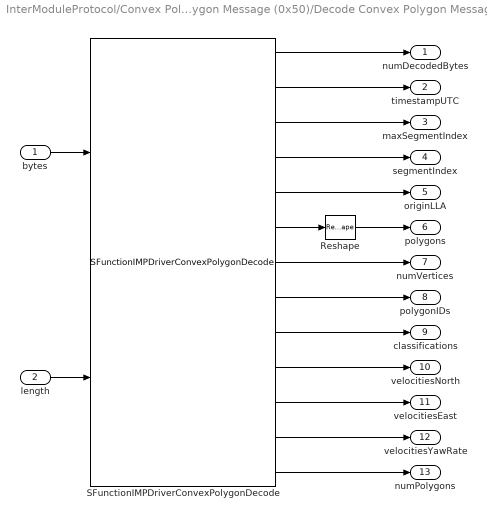
== system InterModuleProtocol/Convex Polygon Message (0x50)/Decode Convex Polygon Message ==
  bytes : Inport  OutDataTypeStr=uint8
  length : Inport  Port=2  OutDataTypeStr=uint32  PortDimensions=1
  Reshape : Reshape  OutputDimensionality=Customize  OutputDimensions=[2,255,maxNumPolygons]
  SFunctionIMPDriverConvexPolygonDecode : S-Function  FunctionName=SFunctionIMPDriverConvexPolygonDecode  Parameters=SParameter1, SampleTime  SFunctionDeploymentMode=off  EnableBusSupport=off  mask(Legacy Function){SFunctionSpec=void IMP_OutputDriverConvexPolygonDecode(uint8 u1[], uint32 u2, int32 y1[1], double y2[1], uint8 y3[1], uint8 y4[1], double y5[3], double y6[2*255*p1], uint16 p1, uint8 y7[p1], uint16 y8[p1], uint8 y9[p1], double y10[p1], double y11[p1], double y12[p1], uint16 y13[1]), SParameter1=uint16(reshape(maxNumPolygons, [1 1])), SampleTime=-1, ShowSpec=off}
      mask prompts: SParameter1 "P1:"; SampleTime "Sample time (-1 for inherited):"; ShowSpec "Display function specification"
      mask help:
      | This block allows you to call the legacy functions specified by the following Legacy Code Tool definition:
      | def.SFunctionName = 'SFunctionIMPDriverConvexPolygonDecode';
      | def.OutputFcnSpec = 'void IMP_OutputDriverConvexPolygonDecode(uint8 u1[], uint32 u2, int32 y1[1], double y2[1], uint8 y3[1], uint8 y4[1], double y5[3], double y6[2*255*p1], uint16 p1, uint8 y7[p1], uint16 y8[p1], uint8 y9[p1], double y10[p1], double y11[p1], double y12[p1], uint16 y13[1])';
      | def.StartFcnSpec = 'void IMP_CreateDriverConvexPolygonDecode()';
      | def.TerminateFcnSpec = 'void IMP_DeleteDriverConvexPolygonDecode()';
      | def.HeaderFiles = {'IMP_DriverConvexPolygonDecode.h'};
      | def.SourceFiles = {'IMP_DriverConvexPolygonDecode.cpp', 'InterModuleProtocol.cpp', 'IMPConvexPolygon.cpp', 'IMPState.cpp', 'IMPStateConfiguration.cpp'};
      | def.IncPaths = {'..\..\source\InterModuleProtocol'};
      | def.SrcPaths = {'..\..\source\InterModuleProtocol'};
      | def.SampleTime = 'parameterized';
      | def.Options.useTlcWithAccel = false;
      mask Help: <p>This block was generated automatically by the Legacy Code Tool. For detailed help on this tool, call<a href="matlab:legacy_code('help')"> legacy_code('help')</a>.</p>
      mask Callback ShowSpec:
      | if strcmp(get_param(gcbh, 'ShowSpec'), 'on')
      |   set_param(gcbh, 'MaskDisplay', sprintf('fprintf(''%s'');', get_param(gcbh, 'SFunctionSpec')));
      | else
      |   set_param(gcbh, 'MaskDisplay', sprintf('fprintf(''%s'');', get_param(gcbh, 'FunctionName')));
      | end
      mask Display: fprintf('SFunctionIMPDriverConvexPolygonDecode');
  numDecodedBytes : Outport  OutDataTypeStr=int32  PortDimensions=1  VectorParamsAs1DForOutWhenUnconnected=off
  timestampUTC : Outport  Port=2  OutDataTypeStr=double  Unit=s  PortDimensions=1  VectorParamsAs1DForOutWhenUnconnected=off
  maxSegmentIndex : Outport  Port=3  OutDataTypeStr=uint8  PortDimensions=1  VectorParamsAs1DForOutWhenUnconnected=off
  segmentIndex : Outport  Port=4  OutDataTypeStr=uint8  PortDimensions=1  VectorParamsAs1DForOutWhenUnconnected=off
  originLLA : Outport  Port=5  OutDataTypeStr=double  PortDimensions=3  VectorParamsAs1DForOutWhenUnconnected=off
  polygons : Outport  Port=6  OutDataTypeStr=double  Unit=m  PortDimensions=[2, 255, maxNumPolygons]  VectorParamsAs1DForOutWhenUnconnected=off
  numVertices : Outport  Port=7  OutDataTypeStr=uint8  PortDimensions=maxNumPolygons  VectorParamsAs1DForOutWhenUnconnected=off
  polygonIDs : Outport  Port=8  OutDataTypeStr=uint16  PortDimensions=maxNumPolygons  VectorParamsAs1DForOutWhenUnconnected=off
  classifications : Outport  Port=9  OutDataTypeStr=uint8  PortDimensions=maxNumPolygons  VectorParamsAs1DForOutWhenUnconnected=off
  velocitiesNorth : Outport  Port=10  OutDataTypeStr=double  Unit=m/s  PortDimensions=maxNumPolygons  VectorParamsAs1DForOutWhenUnconnected=off
  velocitiesEast : Outport  Port=11  OutDataTypeStr=double  Unit=m/s  PortDimensions=maxNumPolygons  VectorParamsAs1DForOutWhenUnconnected=off
  velocitiesYawRate : Outport  Port=12  OutDataTypeStr=double  Unit=rad/s  PortDimensions=maxNumPolygons  VectorParamsAs1DForOutWhenUnconnected=off
  numPolygons : Outport  Port=13  OutDataTypeStr=uint16  PortDimensions=1  VectorParamsAs1DForOutWhenUnconnected=off
  wires:
  bytes/1 -> SFunctionIMPDriverConvexPolygonDecode/1
  length/1 -> SFunctionIMPDriverConvexPolygonDecode/2
  Reshape/1 -> polygons/1
  SFunctionIMPDriverConvexPolygonDecode/1 -> numDecodedBytes/1
  SFunctionIMPDriverConvexPolygonDecode/2 -> timestampUTC/1
  SFunctionIMPDriverConvexPolygonDecode/3 -> maxSegmentIndex/1
  SFunctionIMPDriverConvexPolygonDecode/4 -> segmentIndex/1
  SFunctionIMPDriverConvexPolygonDecode/5 -> originLLA/1
  SFunctionIMPDriverConvexPolygonDecode/6 -> Reshape/1
  SFunctionIMPDriverConvexPolygonDecode/7 -> numVertices/1
  SFunctionIMPDriverConvexPolygonDecode/8 -> polygonIDs/1
  SFunctionIMPDriverConvexPolygonDecode/9 -> classifications/1
  SFunctionIMPDriverConvexPolygonDecode/10 -> velocitiesNorth/1
  SFunctionIMPDriverConvexPolygonDecode/11 -> velocitiesEast/1
  SFunctionIMPDriverConvexPolygonDecode/12 -> velocitiesYawRate/1
  SFunctionIMPDriverConvexPolygonDecode/13 -> numPolygons/1

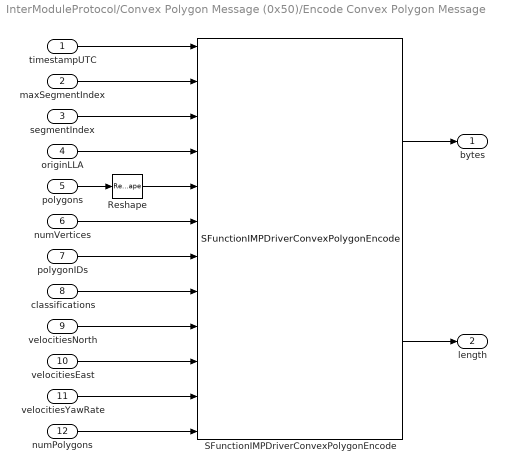
== system InterModuleProtocol/Convex Polygon Message (0x50)/Encode Convex Polygon Message ==
  timestampUTC : Inport  OutDataTypeStr=double  Unit=s  PortDimensions=1
  maxSegmentIndex : Inport  Port=2  OutDataTypeStr=uint8  PortDimensions=1
  segmentIndex : Inport  Port=3  OutDataTypeStr=uint8  PortDimensions=1
  originLLA : Inport  Port=4  OutDataTypeStr=double  PortDimensions=3
  polygons : Inport  Port=5  OutDataTypeStr=double  Unit=m  PortDimensions=[2, 255, maxNumPolygons]
  numVertices : Inport  Port=6  OutDataTypeStr=uint8  PortDimensions=maxNumPolygons
  polygonIDs : Inport  Port=7  OutDataTypeStr=uint16  PortDimensions=maxNumPolygons
  classifications : Inport  Port=8  OutDataTypeStr=uint8  PortDimensions=maxNumPolygons
  velocitiesNorth : Inport  Port=9  OutDataTypeStr=double  Unit=m/s  PortDimensions=maxNumPolygons
  velocitiesEast : Inport  Port=10  OutDataTypeStr=double  Unit=m/s  PortDimensions=maxNumPolygons
  velocitiesYawRate : Inport  Port=11  OutDataTypeStr=double  Unit=rad/s  PortDimensions=maxNumPolygons
  numPolygons : Inport  Port=12  OutDataTypeStr=uint16  PortDimensions=1
  Reshape : Reshape  OutputDimensionality=Customize  OutputDimensions=[2*255*maxNumPolygons,1]
  SFunctionIMPDriverConvexPolygonEncode : S-Function  FunctionName=SFunctionIMPDriverConvexPolygonEncode  Parameters=SParameter1, SParameter2, SampleTime  SFunctionDeploymentMode=off  EnableBusSupport=off  mask(Legacy Function){SFunctionSpec=void IMP_OutputDriverConvexPolygonEncode(uint8 y1[p1], uint32 y2[1], uint32 p1, double u1, uint8 u2, uint8 u3, double u4[3], double u5[2*255*p2], uint16 p2, uint8 u6[p2], uint16 u7[p2], uint8 u8[p2], double u9[p2], double u10[p2], double u11[p2], uint16 u12), SParameter1=uint32(reshape(outBufferSize, [1 1])), SParameter2=uint16(reshape(maxNumPolygons, [1 1])), SampleTime=-1, ShowSpec=off}
      mask prompts: SParameter1 "P1:"; SParameter2 "P2:"; SampleTime "Sample time (-1 for inherited):"; ShowSpec "Display function specification"
      mask help:
      | This block allows you to call the legacy functions specified by the following Legacy Code Tool definition:
      | def.SFunctionName = 'SFunctionIMPDriverConvexPolygonEncode';
      | def.OutputFcnSpec = 'void IMP_OutputDriverConvexPolygonEncode(uint8 y1[p1], uint32 y2[1], uint32 p1, double u1, uint8 u2, uint8 u3, double u4[3], double u5[2*255*p2], uint16 p2, uint8 u6[p2], uint16 u7[p2], uint8 u8[p2], double u9[p2], double u10[p2], double u11[p2], uint16 u12)';
      | def.StartFcnSpec = 'void IMP_CreateDriverConvexPolygonEncode()';
      | def.TerminateFcnSpec = 'void IMP_DeleteDriverConvexPolygonEncode()';
      | def.HeaderFiles = {'IMP_DriverConvexPolygonEncode.h'};
      | def.SourceFiles = {'IMP_DriverConvexPolygonEncode.cpp', 'InterModuleProtocol.cpp', 'IMPConvexPolygon.cpp', 'IMPState.cpp', 'IMPStateConfiguration.cpp'};
      | def.IncPaths = {'..\..\source\InterModuleProtocol'};
      | def.SrcPaths = {'..\..\source\InterModuleProtocol'};
      | def.SampleTime = 'parameterized';
      | def.Options.useTlcWithAccel = false;
      mask Help: <p>This block was generated automatically by the Legacy Code Tool. For detailed help on this tool, call<a href="matlab:legacy_code('help')"> legacy_code('help')</a>.</p>
      mask Callback ShowSpec:
      | if strcmp(get_param(gcbh, 'ShowSpec'), 'on')
      |   set_param(gcbh, 'MaskDisplay', sprintf('fprintf(''%s'');', get_param(gcbh, 'SFunctionSpec')));
      | else
      |   set_param(gcbh, 'MaskDisplay', sprintf('fprintf(''%s'');', get_param(gcbh, 'FunctionName')));
      | end
      mask Display: fprintf('SFunctionIMPDriverConvexPolygonEncode');
  bytes : Outport  OutDataTypeStr=uint8  PortDimensions=outBufferSize  VectorParamsAs1DForOutWhenUnconnected=off
  length : Outport  Port=2  OutDataTypeStr=uint32  PortDimensions=1  VectorParamsAs1DForOutWhenUnconnected=off
  wires:
  polygons/1 -> Reshape/1
  SFunctionIMPDriverConvexPolygonEncode/1 -> bytes/1
  SFunctionIMPDriverConvexPolygonEncode/2 -> length/1
  timestampUTC/1 -> SFunctionIMPDriverConvexPolygonEncode/1
  maxSegmentIndex/1 -> SFunctionIMPDriverConvexPolygonEncode/2
  segmentIndex/1 -> SFunctionIMPDriverConvexPolygonEncode/3
  originLLA/1 -> SFunctionIMPDriverConvexPolygonEncode/4
  Reshape/1 -> SFunctionIMPDriverConvexPolygonEncode/5
  numVertices/1 -> SFunctionIMPDriverConvexPolygonEncode/6
  polygonIDs/1 -> SFunctionIMPDriverConvexPolygonEncode/7
  numPolygons/1 -> SFunctionIMPDriverConvexPolygonEncode/12
  classifications/1 -> SFunctionIMPDriverConvexPolygonEncode/8
  velocitiesNorth/1 -> SFunctionIMPDriverConvexPolygonEncode/9
  velocitiesEast/1 -> SFunctionIMPDriverConvexPolygonEncode/10
  velocitiesYawRate/1 -> SFunctionIMPDriverConvexPolygonEncode/11
